simulink model "eTimer_measure"  (R2018a)
settings: Solver=FixedStepDiscrete  StartTime=0.0  StopTime=50  FixedStep=1  RelTol=1e-3  EnableMultiTasking=on
InitFcn:
  | mbd_pnt_consistency_checks(bdroot(gcs));
undefined symbols (not defined in the file): A11, D10
libraries: mbd_pnt_ec_toolbox x4
Description:
  | This model shows how to measure the PWM signal period with eTimer
  | 
  | The FlexPWM module 0, submodule 0, is configured to generated a PWM waveform
  | on A10 and A11 pins (J1.5 and J1.7). The frequency is changing @5sec between
  | 1000Hz and 10000Hz
  | 
  | The eTimer is configured to read the signal from A0 (J5.1)
  | 
  | Connect a wire between any of J1.5/J1.7 and J5.1 to have meaningfull data.
settings Model: Creator=vkostrov  LastModifiedBy=oolonthegreat
settings DataIOCC: ExternalInput=off  InitialState=off  LimitDataPoints=on  SaveFormat=Array  SignalLoggingSaveFormat=ModelDataLogs  SaveOutput=off  SignalLogging=off  SaveTime=off
settings OptimizationCC: DefaultParameterBehavior=Inlined  ExpressionDepthLimit=2147483647  LifeSpan=1
settings DebuggingCC: UnderspecifiedInitializationDetection=Classic  MergeDetectMultiDrivingBlocksExec=none  SolverPrmCheckMsg=warning  InheritedTsInSrcMsg=none  SingleTaskRateTransMsg=error  FcnCallInpInsideContextMsg=warning  UnconnectedInputMsg=error  UnconnectedOutputMsg=error  UnconnectedLineMsg=error  AllowSymbolicDim=off  UnknownTsInhSupMsg=error  StateNameClashWarn=warning  SFUnexpectedBacktrackingDiag=warning  SFNoUnconditionalDefaultTransitionDiag=warning  SFExecutionAtInitializationDiag=none
settings HardwareCC: ProdBitPerPointer=32  ProdBitPerSizeT=32  ProdBitPerPtrDiffT=32  ProdLargestAtomicInteger=Long  ProdLargestAtomicFloat=Double  ProdEndianess=BigEndian  ProdWordSize=32  ProdHWDeviceType=Motorola PowerPC
settings ModelReferenceCC: PropagateSignalLabelsOutOfModel=off
settings SFSimCC: MATLABDynamicMemAlloc=off
settings RTWCC: SystemTargetFile=mbd_pnt.tlc  MakeCommand=mbd_pnt_make_rtw COPY_MDLREF_INCLUDES=0  TemplateMakefile=mbd_pnt.tmf  PostCodeGenCommand=mbd_pnt_analyzegencode(buildInfo)  Description=Model Based Design Toolbox MPC574xP Code Generation Target
settings CodeAppCC: IgnoreCustomStorageClasses=off  CustomSymbolStrType=$N$R$M  StateflowObjectComments=on  InternalIdentifier=Classic
settings STFCustomTargetCC: CombineOutputUpdateFcns=on  SuppressErrorStatus=on  ERTCustomFileBanners=on  SupportContinuousTime=off  SupportNonInlinedSFcns=off  RemoveResetFunc=on  MATLABClassNameForMDSCustomization=Simulink.SoftwareTarget.ERTCustomization  GRTInterface=off  SystemTargetFile=mbd_pnt.tlc
settings ERTTargetCC: MultiwordLength=2048  ParMdlRefBuildCompliant=off  CompOptLevelCompliant=off  ConcurrentExecutionCompliant=off  SuppressErrorStatus=on  ModelStepFunctionPrototypeControlCompliant=off  CPPClassGenCompliant=off  UseToolchainInfoCompliant=off  ExtModeMexFile=noextcomm  InlinedParameterPlacement=NonHierarchical  ERTCustomFileTemplate=example_file_process.tlc  ConvertIfToSwitch=off  SuppressUnreachableDefaultCases=off
settings ConfigComp: CovMetricSettings=dw  CovHtmlReporting=on  CovSaveCumulativeToWorkspaceVar=on  CovSaveSingleToWorkspaceVar=on  CovExternalEMLEnable=off

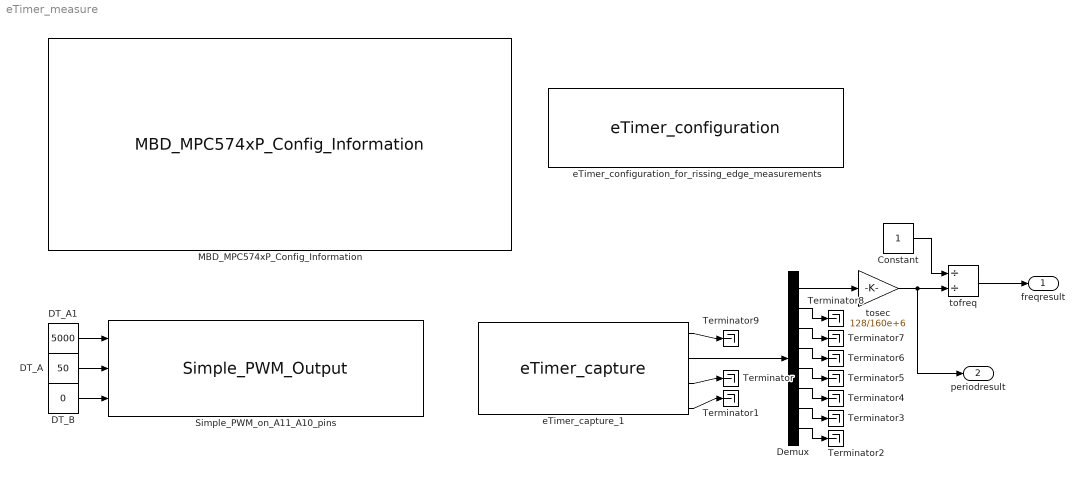
== system eTimer_measure ==
  Constant : Constant  OutDataTypeStr=uint16
  DT_A : Constant  Value=50  OutDataTypeStr=uint32
  DT_A1 : Constant  Value=5000  OutDataTypeStr=uint32
  DT_B : Constant  Value=0  OutDataTypeStr=uint32
  Demux : Demux  Outputs=8
  MBD_MPC574xP_Config_Information : mbd_pnt_ec_toolbox/MPC574xP/MBD_MPC574xP_Config_Information  disp_str=|  config_params=[]
      | System Clock : 200 MHz
      | Target : MPC5744P
      | Package : 144LQFP
      | XTAL Freq : 40 MHz
      | Compiler : S32 Design Studio
      | Target Type : FLASH
      | Global Interrupt Priority : 8
      | System Tick Interrupt Priority : 12
      | Freemaster : Serial1 (115200 Kbits)
      | Download Code after build : (COM5,115200)
      settings: SourceProductName=Model Based Design Toolbox for MPC574xP
  Simple_PWM_on_A11_A10_pins : mbd_pnt_ec_toolbox/MPC574xP/Motor Control Blocks/Simple_PWM_Output  pwmModule=0  pwmMod=0  SubModule=0  subMod=0  InitFreq=1000  resolution=1 %  resValue=1  InitDutyA=0  InitDutyB=0  align=edge aligned  PhaseShift_A=0  PhaseShift_B=0  Phase_A=0  Phase_B=0  centered=0  doubleSw=off  DoubleS=0  debugSw=off  debug_mode=0  pin0_A0=11: A11 : [120] : [149] : [D10]  pin0_B0=None  pin0_X0=None  pin0_A1=None  pin0_B1=None  pin0_X1=None  pin0_A2=None  pin0_B2=None  pin0_X2=None  pin0_A3=None  pin0_B3=None  pin0_X3=None  pin1_A0=None  pin1_B0=None  pin1_X0=None  pin1_A1=None  pin1_B1=None  pin1_X1=None  pin1_A2=None  pin1_B2=None  pin1_X2=None  pin1_A3=None  pin1_B3=None  pin1_X3=None  pin2_A0=None  pin2_B0=None  pin2_X0=None  pin2_A1=None  pin2_B1=None  pin2_X1=None  pin2_A2=None  pin2_B2=None  pin2_X2=None  pin2_A3=None  pin2_B3=None  pin2_X3=None  pcrNumA=11  pcrNumB=255  pcrNumX=255  polA=off  polB=off  polX=off  octrl=0  syncFrom0=off  masterSync=0  outVal0=off  outVal1=off  outVal2=off  outVal3=off  outVal4=off  outVal5=off  outTrig=0
      settings: SourceProductName=Model Based Design Toolbox for MPC574xP
  Terminator{,1..9} (10 alike) : Terminator
  eTimer_capture_1 : mbd_pnt_ec_toolbox/MPC574xP/Motor Control Blocks/eTimer_capture  SubModule=0  Timerchan=0  subMod=0  channel=0
      settings: SourceProductName=Model Based Design Toolbox for MPC574xP
  eTimer_configuration_for_rissing_edge_measurements : mbd_pnt_ec_toolbox/MPC574xP/Motor Control Blocks/eTimer_configuration  SubModule=0  TimerChan=0  subMod=0  channel=0  CountMode=001 - Count rising edges of primary source  CNTMODE=1  CountOnce=0 - Count repeatedly  ONCE=0  CountLength=0 - Continue counting to roll over  LENGTH=0  CountDirection=0 - Count up  DIR=0  OutputEnable=0 - The external pin is configured as an input  OEN=0  CoChanInit=00 - Other channels cannot force re-initialization of this channel  COINIT=0  StopAction=0 - Output enable is unaffected by stop mode  STPEN=0  ReloadOnCapt=01 - Reload the counter on a capture 1 event  ROC=1  PrimarySource=11111 - IP Bus clock divide by 128 prescaler  PRISRC=31  PrimSrcPol=0 - True polarity  PIPS=0  SecondarySource=00000 - Counter #0 input pin  SECSRC=0  SecSrcPol=0 - True polarity  SIPS=0  FILT_CNT=0  FILT_PER=0  FILT=0  OutputMode=0000 - Software controlled  OUTMODE=0  OutputPol=0 - True polarity  OPS=0  MasterMode=0 - Disable broadcast of this channel output  MSTR=0  ForcedOutVal=0  VAL=0  CoForce=0 - Other channels cannot force this channel output  COFRC=0  CompLoad1=000 - COMP1 is never preload  CLC1=0  CompLoad2=000 - COMP2 is never preload  CLC2=0  CompareMode="00 - COMP1 and COMP2  are used when the counter is counting up"  CMPMODE=0  CaptMode1=10 - Capture rising edges  CPT1MODE=2  CaptMode2=00 - Capture disabled  CPT2MODE=0  OneShCaptMode=0 - Free running mode is selected  ONESHOT=0  CaptFIFO=0  CFWM=0  CNTRinit=0  COMP1init=0  COMP2init=0  mod0ch0pin="0     : A0   :  [73]   : [86]   : [P12]  input/output"  mod0ch1pin=None  mod0ch2pin=None  mod0ch3pin=None  mod0ch4pin=None  mod0ch5pin=None  mod1ch0pin=None  mod1ch1pin=None  mod1ch2pin=None  mod1ch3pin=None  mod1ch4pin=None  mod1ch5pin=None  mod2ch0pin=None  mod2ch1pin=None  mod2ch2pin=None  mod2ch3pin=None  mod2ch4pin=None  mod2ch5pin=None  pcrNum0=0  pcrNum1=255  pcrNum2=255  pcrNum3=255  pcrNum4=255  pcrNum5=255  TCFIE=off  TCF1IE=off  TCF2IE=off  TOFIE=off  IELFIE=off  IEHFIE=off  ICF1IE=off  ICF2IE=off  INTDMA=0
      settings: SourceProductName=Model Based Design Toolbox for MPC574xP
  tofreq : Product  Inputs=//  OutDataTypeStr=uint16
  tosec : Gain  Gain=128/160e+6  OutDataTypeStr=single
  freqresult : Outport
  periodresult : Outport  Port=2
  wires:
  DT_A1/1 -> Simple_PWM_on_A11_A10_pins/1
  DT_A/1 -> Simple_PWM_on_A11_A10_pins/2
  DT_B/1 -> Simple_PWM_on_A11_A10_pins/3
  eTimer_capture_1/2 -> Demux/1
  eTimer_capture_1/3 -> Terminator/1
  eTimer_capture_1/4 -> Terminator1/1
  Demux/8 -> Terminator2/1
  Demux/7 -> Terminator3/1
  Demux/6 -> Terminator4/1
  Demux/5 -> Terminator5/1
  Demux/4 -> Terminator6/1
  Demux/3 -> Terminator7/1
  Demux/2 -> Terminator8/1
  Demux/1 -> tosec/1
  eTimer_capture_1/1 -> Terminator9/1
  Constant/1 -> tofreq/1
  tosec/1 -> periodresult/1, tofreq/2
  tofreq/1 -> freqresult/1
